simulink model "js_Lcontroller"  (R2017b)
settings: Solver=VariableStepAuto  StartTime=0.0  StopTime=10.0  RelTol=1e-3
settings Model: Creator=Kalana  LastModifiedBy=Kalana

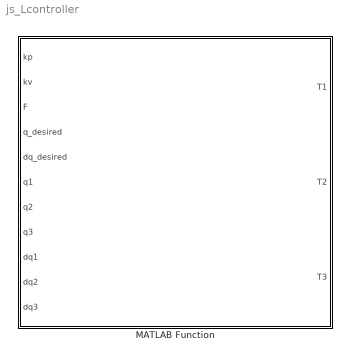
== system js_Lcontroller ==
  MATLAB Function : MATLAB Function  TreatAsAtomicUnit=on

== matlab function js_Lcontroller/MATLAB Function ==
  data: kp input; kv input; F input; T1 output; q_desired input; dq_desired input; q1 input; T2 output; T3 output; q2 input; q3 input; dq1 input; dq2 input; dq3 input
function [T1, T2, T3]  = leftLegControl(kp, kv, F, q_desired, dq_desired, q1, q2, q3, dq1, dq2, dq3)

g = [0    ;
     0    ;
     -9.8 ];
 
q = [q1; 
     q2; 
     q3];
 
dq = [dq1; 
      dq2;
      dq3];

Mass_1 = [1.14619,  0,        0;
          0,        1.14619,  0;
          0,        0,        1.14619];

Iner_1 = [ 4703123.40e-09,      3169987.54e-09,     -298.39e-09;
           3169987.54e-09,      4976200.05e-09,     -448.10e-09;
           -298.39e-09,         -448.10e-09,         8601987.18e-09];

      
Mass_2 = [1.14271,  0,        0;
          0,        1.14271,  0;
          0,        0,        1.14271];

Iner_2 = [2565669.28e-09,     -227.65e-09,          -2839719.99e-09;
           -227.65e-09,        12592910.15e-09,     9.39e-09;
          -2839719.99e-09,     9.39e-09,            10643970.45e-09];

      
Mass_3 = [0.63820,  0,        0;
          0,        0.63820,  0;
          0,        0,        0.63280];
  
Iner_3 = [728680.81e-09,      -172.39e-09,        158.48e-09;
          -172.39e-09,        2618699.35e-09,     -3.33e-09;
          158.48e-09,         -3.33e-09,          2391085.66e-09];

      
Jv1 = [0.05734*cosd(q1)-0.05586*sind(q1),    0, 0;
       0,                                    0, 0;
       -0.05734*sind(q1)-0.05586*cosd(q1)    0, 0];

Jw1 = [0, 0, 0;
       1, 0, 0;
       0, 0, 0];

   
Jv2 = [-0.100*sind(q1)*cosd(q2)-0.02771*cosd(q1)-0.1225*sind(q1),  -0.100*cosd(q1)*sind(q2),     0;
       0,                                                          0.100*cosd(q2),               0; 
       0.100*cosd(q1)*cosd(q2)+0.02771*sind(q1)-0.1225*cosd(q1),   -0.100*sind(q1)*sind(q2),     0]; 
      
Jw2 = [0, 1, 0; 
       1, 0, 0; 
       0, 0, 0];
 
   
Jv3 = [-0.02559*sind(q1)*cosd(q2-q3)-0.2*sind(q1)*cosd(q2)-0.1225*sind(q1)-0.0525*cosd(q1),  -0.02559*cosd(q1)*sind(q2-q3)-0.2*cosd(q1)*sind(q2),  0.02559*cosd(q1)*sind(q2-q3) ;
       0,                                                                                    0.02559*cosd(q2-q3)+0.2*cosd(q2),                     -0.02559*cosd(q2-q3)         ;
       -0.02559*cosd(q1)*cosd(q2-q3)-0.2*cosd(q1)*cosd(q2)-0.1225*cosd(q1)+0.0525*sind(q1),  0.02559*sind(q1)*sind(q2-q3)+0.2*sind(q1)*sind(q2),   -0.02559*sind(q1)*sind(q2-q3)];
      
Jw3 = [0, 1, -1;
       1, 0,  0;
       0, 0,  0];

   
JvEE =[-0.265*sind(q1)*cosd(q2-q3)-0.2*sind(q1)*cosd(q2)-0.1225*sind(q1)-0.0525*cosd(q1), -0.265*cosd(q1)*sind(q2-q3)-0.2*cosd(q1)*sind(q2),     0.265*cosd(q1)*sind(q2-q3) ;
       0,                                                                                 0.265*cosd(q2-q3)+0.2*cosd(q2),                        -0.265*cosd(q2-q3)         ;
       -0.265*cosd(q1)*cosd(q2-q3)-0.2*cosd(q1)*cosd(q2)-0.1225*cosd(q1)+0.0525*sind(q1), 0.265*sind(q1)*sind(q2-q3)+0.2*sind(q1)*sind(q2),      -0.265*sind(q1)*sind(q2-q3)]; 
  

Mass = Jv1'*Mass_1*Jv1 + Jw1'*Iner_1*Jw1 + Jv2'*Mass_2*Jv2 + Jw2'*Iner_2*Jw2 + Jv3'*Mass_3*Jv3 + Jw3'*Iner_3*Jw3;

Grav = Jv1'*M1*g + Jv2'*M2*g + Jv3'*M3*g;

Force = JvEE'*F;

torque = Mass(kp(q_desired - q) + kv(dq_desired - qd)) + Grav + Force;

T1 = torque(1);
T2 = torque(2);
T3 = torque(3)
